simulink model "dl_adaptor"  (R2020b)
settings: Solver=ode45  StartTime=0.0  StopTime=sim_time  RelTol=1e-3  EnableMultiTasking=on
values from neighbouring files (symbols this model uses):
  bw_case = 0    [dl_adaptor_init.m]
  compression_mode = 0    [dl_adaptor_init.m]
  data_bin_pt = 0    [dl_adaptor_init.m]
  data_bit_width = 16    [dl_adaptor_init.m]
  dl_oran_gain_bin_pt = 14    [dl_adaptor_init.m]
  dl_oran_gain_reg = round(dl_oran_gain_reg*2^dl_oran_gain_bin_pt)*2^-dl_oran_gain_bin_pt    [dl_adaptor_init.m]
  eq_gain_bit_width = 9    [dl_adaptor_init.m]
  equalization_bypass = 0    [dl_adaptor_init.m]
  gain_bit_width = 16    [dl_adaptor_init.m]
  IQ_exp_offset = 0    [dl_adaptor_init.m]
  RAT_mode = 0    [dl_adaptor_init.m]
  sys_clk = 491.52e6    (= 491520000)    [dl_adaptor_init.m]
undefined symbols (not defined in the file or in its folder): A, A2, B, D, i, W, X, Z
libraries: xbsIndex_r4 x372
(part 2 of 2)

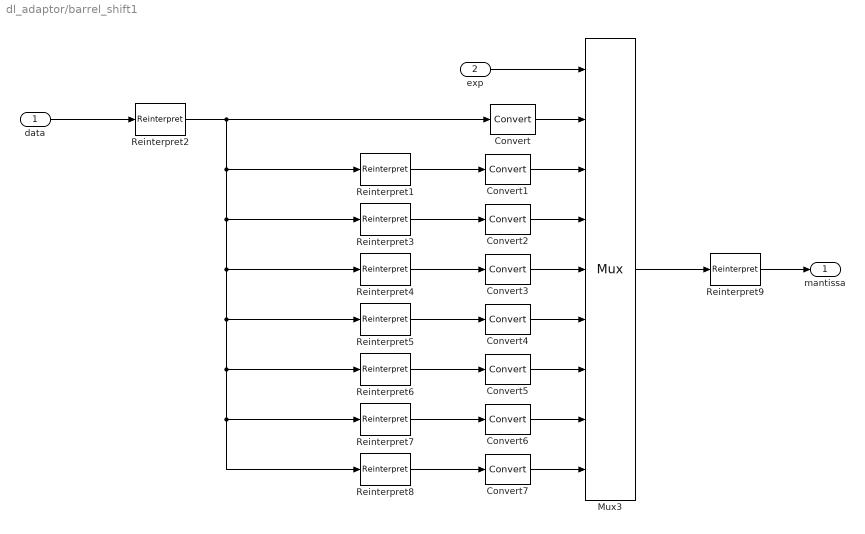
== system dl_adaptor/barrel_shift1 ==
  data : Inport
  exp : Inport  Port=2
  Convert{,1..7} (8 alike) : xbsIndex_r4/Convert  gui_display_data_type=Fixed-point  arith_type="Signed  (2's comp)"  n_bits=data_bit_width  bin_pt=7  float_type=Single  exp_bits=8  fraction_bits=24  quantization=Truncate  overflow=Wrap  en=off  latency=0  pipeline=off  dbl_ovrd=off  block_type=convert
  Mux3 : xbsIndex_r4/Mux  inputs=8  en=off  latency=0  precision=Full  arith_type=Unsigned  n_bits=16  bin_pt=14  quantization=Truncate  overflow=Wrap  dbl_ovrd=off  block_type=mux
  Reinterpret1 : xbsIndex_r4/Reinterpret  force_arith_type=on  arith_type="Signed  (2's comp)"  force_bin_pt=on  bin_pt=6  block_type=reinterpret
  Reinterpret2 : xbsIndex_r4/Reinterpret  force_arith_type=on  arith_type="Signed  (2's comp)"  force_bin_pt=on  bin_pt=7  block_type=reinterpret
  Reinterpret3 : xbsIndex_r4/Reinterpret  force_arith_type=on  arith_type="Signed  (2's comp)"  force_bin_pt=on  bin_pt=5  block_type=reinterpret
  Reinterpret4 : xbsIndex_r4/Reinterpret  force_arith_type=on  arith_type="Signed  (2's comp)"  force_bin_pt=on  bin_pt=4  block_type=reinterpret
  Reinterpret5 : xbsIndex_r4/Reinterpret  force_arith_type=on  arith_type="Signed  (2's comp)"  force_bin_pt=on  bin_pt=3  block_type=reinterpret
  Reinterpret6 : xbsIndex_r4/Reinterpret  force_arith_type=on  arith_type="Signed  (2's comp)"  force_bin_pt=on  bin_pt=2  block_type=reinterpret
  Reinterpret7 : xbsIndex_r4/Reinterpret  force_arith_type=on  arith_type="Signed  (2's comp)"  force_bin_pt=on  bin_pt=1  block_type=reinterpret
  Reinterpret8 : xbsIndex_r4/Reinterpret  force_arith_type=on  arith_type="Signed  (2's comp)"  force_bin_pt=on  bin_pt=0  block_type=reinterpret
  Reinterpret9 : xbsIndex_r4/Reinterpret  force_arith_type=on  arith_type="Signed  (2's comp)"  force_bin_pt=on  bin_pt=0  block_type=reinterpret
  mantissa : Outport  VectorParamsAs1DForOutWhenUnconnected=off
  wires:
  data/1 -> Reinterpret2/1
  Reinterpret1/1 -> Convert1/1
  exp/1 -> Mux3/1
  Mux3/1 -> Reinterpret9/1
  Convert/1 -> Mux3/2
  Convert1/1 -> Mux3/3
  Convert2/1 -> Mux3/4
  Convert3/1 -> Mux3/5
  Convert4/1 -> Mux3/6
  Convert5/1 -> Mux3/7
  Convert6/1 -> Mux3/8
  Reinterpret2/1 -> Convert/1, Reinterpret1/1, Reinterpret3/1, Reinterpret4/1, Reinterpret5/1, Reinterpret6/1, Reinterpret8/1, Reinterpret7/1
  Convert7/1 -> Mux3/9
  Reinterpret3/1 -> Convert2/1
  Reinterpret4/1 -> Convert3/1
  Reinterpret5/1 -> Convert4/1
  Reinterpret6/1 -> Convert5/1
  Reinterpret7/1 -> Convert6/1
  Reinterpret8/1 -> Convert7/1
  Reinterpret9/1 -> mantissa/1

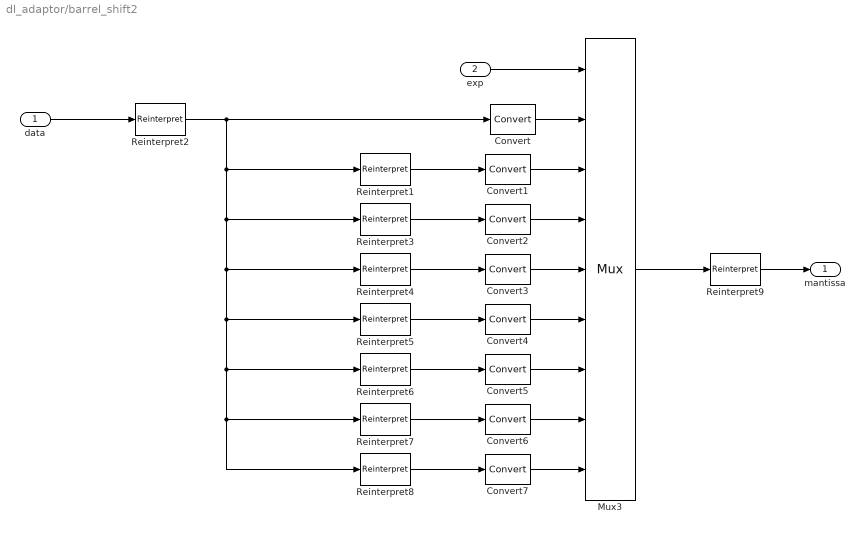
== system dl_adaptor/barrel_shift2 ==
  data : Inport
  exp : Inport  Port=2
  Convert{,1..7} (8 alike) : xbsIndex_r4/Convert  gui_display_data_type=Fixed-point  arith_type="Signed  (2's comp)"  n_bits=data_bit_width  bin_pt=7  float_type=Single  exp_bits=8  fraction_bits=24  quantization=Truncate  overflow=Wrap  en=off  latency=0  pipeline=off  dbl_ovrd=off  block_type=convert
  Mux3 : xbsIndex_r4/Mux  inputs=8  en=off  latency=0  precision=Full  arith_type=Unsigned  n_bits=16  bin_pt=14  quantization=Truncate  overflow=Wrap  dbl_ovrd=off  block_type=mux
  Reinterpret1 : xbsIndex_r4/Reinterpret  force_arith_type=on  arith_type="Signed  (2's comp)"  force_bin_pt=on  bin_pt=6  block_type=reinterpret
  Reinterpret2 : xbsIndex_r4/Reinterpret  force_arith_type=on  arith_type="Signed  (2's comp)"  force_bin_pt=on  bin_pt=7  block_type=reinterpret
  Reinterpret3 : xbsIndex_r4/Reinterpret  force_arith_type=on  arith_type="Signed  (2's comp)"  force_bin_pt=on  bin_pt=5  block_type=reinterpret
  Reinterpret4 : xbsIndex_r4/Reinterpret  force_arith_type=on  arith_type="Signed  (2's comp)"  force_bin_pt=on  bin_pt=4  block_type=reinterpret
  Reinterpret5 : xbsIndex_r4/Reinterpret  force_arith_type=on  arith_type="Signed  (2's comp)"  force_bin_pt=on  bin_pt=3  block_type=reinterpret
  Reinterpret6 : xbsIndex_r4/Reinterpret  force_arith_type=on  arith_type="Signed  (2's comp)"  force_bin_pt=on  bin_pt=2  block_type=reinterpret
  Reinterpret7 : xbsIndex_r4/Reinterpret  force_arith_type=on  arith_type="Signed  (2's comp)"  force_bin_pt=on  bin_pt=1  block_type=reinterpret
  Reinterpret8 : xbsIndex_r4/Reinterpret  force_arith_type=on  arith_type="Signed  (2's comp)"  force_bin_pt=on  bin_pt=0  block_type=reinterpret
  Reinterpret9 : xbsIndex_r4/Reinterpret  force_arith_type=on  arith_type="Signed  (2's comp)"  force_bin_pt=on  bin_pt=0  block_type=reinterpret
  mantissa : Outport  VectorParamsAs1DForOutWhenUnconnected=off
  wires:
  data/1 -> Reinterpret2/1
  Reinterpret1/1 -> Convert1/1
  exp/1 -> Mux3/1
  Mux3/1 -> Reinterpret9/1
  Convert/1 -> Mux3/2
  Convert1/1 -> Mux3/3
  Convert2/1 -> Mux3/4
  Convert3/1 -> Mux3/5
  Convert4/1 -> Mux3/6
  Convert5/1 -> Mux3/7
  Convert6/1 -> Mux3/8
  Reinterpret2/1 -> Convert/1, Reinterpret1/1, Reinterpret3/1, Reinterpret4/1, Reinterpret5/1, Reinterpret6/1, Reinterpret8/1, Reinterpret7/1
  Convert7/1 -> Mux3/9
  Reinterpret3/1 -> Convert2/1
  Reinterpret4/1 -> Convert3/1
  Reinterpret5/1 -> Convert4/1
  Reinterpret6/1 -> Convert5/1
  Reinterpret7/1 -> Convert6/1
  Reinterpret8/1 -> Convert7/1
  Reinterpret9/1 -> mantissa/1

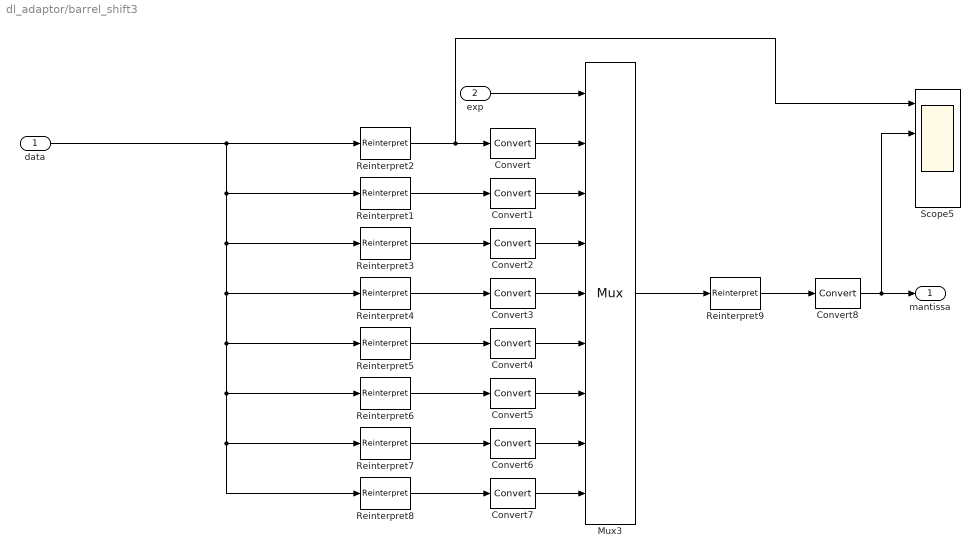
== system dl_adaptor/barrel_shift3 ==
  data : Inport
  exp : Inport  Port=2
  Convert{,1..7} (8 alike) : xbsIndex_r4/Convert  gui_display_data_type=Fixed-point  arith_type=Unsigned  n_bits=gain_bit_width-1  bin_pt=4  float_type=Single  exp_bits=8  fraction_bits=24  quantization=Truncate  overflow=Wrap  en=off  latency=0  pipeline=off  dbl_ovrd=off  block_type=convert
  Convert8 : xbsIndex_r4/Convert  gui_display_data_type=Fixed-point  arith_type="Signed  (2's comp)"  n_bits=gain_bit_width  bin_pt=gain_bin_pt  float_type=Single  exp_bits=8  fraction_bits=24  quantization=Truncate  overflow=Wrap  en=off  latency=0  pipeline=off  dbl_ovrd=off  block_type=convert
  Mux3 : xbsIndex_r4/Mux  inputs=8  en=off  latency=0  precision=Full  arith_type=Unsigned  n_bits=16  bin_pt=14  quantization=Truncate  overflow=Wrap  dbl_ovrd=off  block_type=mux
  Reinterpret1 : xbsIndex_r4/Reinterpret  force_arith_type=on  arith_type=Unsigned  force_bin_pt=on  bin_pt=1  block_type=reinterpret
  Reinterpret2 : xbsIndex_r4/Reinterpret  force_arith_type=on  arith_type=Unsigned  force_bin_pt=on  bin_pt=0  block_type=reinterpret
  Reinterpret3 : xbsIndex_r4/Reinterpret  force_arith_type=on  arith_type=Unsigned  force_bin_pt=on  bin_pt=2  block_type=reinterpret
  Reinterpret4 : xbsIndex_r4/Reinterpret  force_arith_type=on  arith_type=Unsigned  force_bin_pt=on  bin_pt=3  block_type=reinterpret
  Reinterpret5 : xbsIndex_r4/Reinterpret  force_arith_type=on  arith_type=Unsigned  force_bin_pt=on  bin_pt=4  block_type=reinterpret
  Reinterpret6 : xbsIndex_r4/Reinterpret  force_arith_type=on  arith_type=Unsigned  force_bin_pt=on  bin_pt=5  block_type=reinterpret
  Reinterpret7 : xbsIndex_r4/Reinterpret  force_arith_type=on  arith_type=Unsigned  force_bin_pt=on  bin_pt=6  block_type=reinterpret
  Reinterpret8 : xbsIndex_r4/Reinterpret  force_arith_type=on  arith_type=Unsigned  force_bin_pt=on  bin_pt=7  block_type=reinterpret
  Reinterpret9 : xbsIndex_r4/Reinterpret  force_arith_type=on  arith_type=Unsigned  force_bin_pt=on  bin_pt=gain_bit_width-1  block_type=reinterpret
  Scope5 : Scope  NumInputPorts=4
  mantissa : Outport  VectorParamsAs1DForOutWhenUnconnected=off
  wires:
  Reinterpret1/1 -> Convert1/1
  exp/1 -> Mux3/1
  Mux3/1 -> Reinterpret9/1
  Convert/1 -> Mux3/2
  Convert1/1 -> Mux3/3
  Convert2/1 -> Mux3/4
  Convert3/1 -> Mux3/5
  Convert4/1 -> Mux3/6
  Convert5/1 -> Mux3/7
  Convert6/1 -> Mux3/8
  data/1 -> Reinterpret2/1, Reinterpret1/1, Reinterpret3/1, Reinterpret4/1, Reinterpret5/1, Reinterpret6/1, Reinterpret8/1, Reinterpret7/1
  Convert7/1 -> Mux3/9
  Reinterpret3/1 -> Convert2/1
  Reinterpret4/1 -> Convert3/1
  Reinterpret5/1 -> Convert4/1
  Reinterpret6/1 -> Convert5/1
  Reinterpret7/1 -> Convert6/1
  Reinterpret8/1 -> Convert7/1
  Reinterpret9/1 -> Convert8/1
  Reinterpret2/1 -> Scope5/1, Convert/1
  Convert8/1 -> Scope5/2, mantissa/1

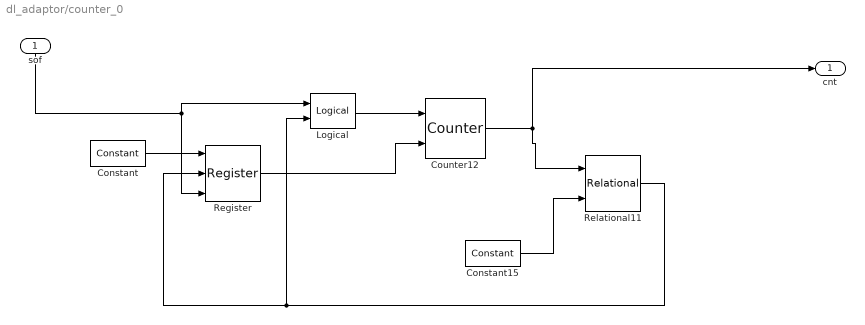
== system dl_adaptor/counter_0 ==
  sof : Inport
  Constant : xbsIndex_r4/Constant  const=1  gui_display_data_type=Boolean  arith_type=Boolean  n_bits=16  bin_pt=14  preci_type=Single  exp_width=8  frac_width=24  explicit_period=off  period=1  equ=P=C  opselect=C  inp2=PCIN>>17  opr=+  inp1=P  carry=CIN  dbl_ovrd=off  block_type=constant
  Constant15 : xbsIndex_r4/Constant  const=2^16-2  gui_display_data_type=Fixed-point  arith_type=Unsigned  n_bits=16  bin_pt=0  preci_type=Single  exp_width=8  frac_width=24  explicit_period=off  period=1  equ=P=C  opselect=C  inp2=PCIN>>17  opr=+  inp1=P  carry=CIN  dbl_ovrd=off  block_type=constant
  Counter12 : xbsIndex_r4/Counter  cnt_type=Free Running  cnt_to=Inf  operation=Up  start_count=0  cnt_by_val=1  arith_type=Unsigned  n_bits=16  bin_pt=0  load_pin=off  rst=on  en=on  explicit_period=on  period=tc  use_behavioral_HDL=off  implementation=Fabric  dbl_ovrd=off  block_type=counter
  Logical : xbsIndex_r4/Logical  logical_function=OR  inputs=2  en=off  latency=0  precision=Full  arith_type=Unsigned  n_bits=16  bin_pt=0  align_bp=on  dbl_ovrd=off  block_type=logical
  Register : xbsIndex_r4/Register  init=0  rst=on  en=on  dbl_ovrd=off  block_type=register
  Relational11 : xbsIndex_r4/Relational  mode=a=b  op_type=Bool  en=off  latency=1  dbl_ovrd=off  block_type=relational
  cnt : Outport  VectorParamsAs1DForOutWhenUnconnected=off
  wires:
  Counter12/1 -> Relational11/1, cnt/1
  Constant15/1 -> Relational11/2
  Register/1 -> Counter12/2
  Constant/1 -> Register/1
  sof/1 -> Logical/1, Register/3
  Logical/1 -> Counter12/1
  Relational11/1 -> Logical/2, Register/2

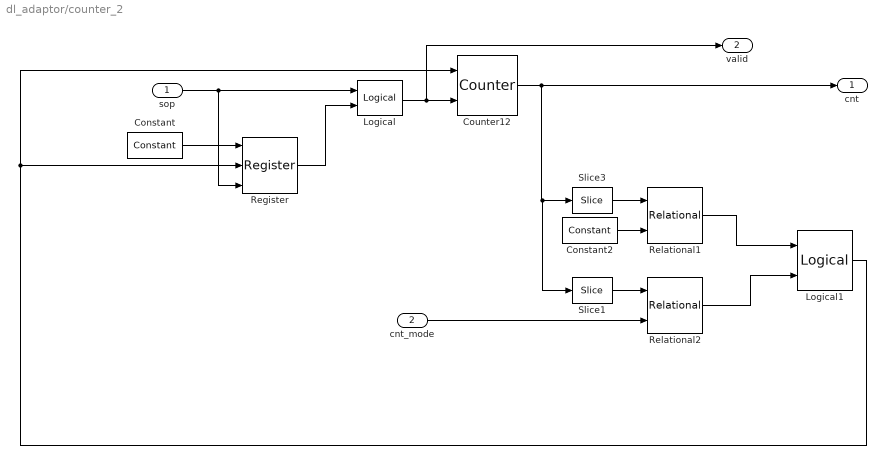
== system dl_adaptor/counter_2 ==
  sop : Inport
  cnt_mode : Inport  Port=2
  Constant : xbsIndex_r4/Constant  const=1  gui_display_data_type=Boolean  arith_type=Boolean  n_bits=16  bin_pt=14  preci_type=Single  exp_width=8  frac_width=24  explicit_period=off  period=1  equ=P=C  opselect=C  inp2=PCIN>>17  opr=+  inp1=P  carry=CIN  dbl_ovrd=off  block_type=constant
  Constant2 : xbsIndex_r4/Constant  const=2^13-2  gui_display_data_type=Fixed-point  arith_type=Unsigned  n_bits=13  bin_pt=0  preci_type=Single  exp_width=8  frac_width=24  explicit_period=off  period=1  equ=P=C  opselect=C  inp2=PCIN>>17  opr=+  inp1=P  carry=CIN  dbl_ovrd=off  block_type=constant
  Counter12 : xbsIndex_r4/Counter  cnt_type=Free Running  cnt_to=Inf  operation=Up  start_count=0  cnt_by_val=1  arith_type=Unsigned  n_bits=15  bin_pt=0  load_pin=off  rst=on  en=on  explicit_period=on  period=tc  use_behavioral_HDL=off  implementation=Fabric  dbl_ovrd=off  block_type=counter
  Logical : xbsIndex_r4/Logical  logical_function=OR  inputs=2  en=off  latency=0  precision=Full  arith_type=Unsigned  n_bits=16  bin_pt=0  align_bp=on  dbl_ovrd=off  block_type=logical
  Logical1 : xbsIndex_r4/Logical  logical_function=AND  inputs=2  en=off  latency=1  precision=Full  arith_type=Unsigned  n_bits=16  bin_pt=0  align_bp=on  dbl_ovrd=off  block_type=logical
  Register : xbsIndex_r4/Register  init=0  rst=on  en=on  dbl_ovrd=off  block_type=register
  Relational1 : xbsIndex_r4/Relational  mode=a=b  op_type=Bool  en=off  latency=0  dbl_ovrd=off  block_type=relational
  Relational2 : xbsIndex_r4/Relational  mode=a=b  op_type=Bool  en=off  latency=0  dbl_ovrd=off  block_type=relational
  Slice1 : xbsIndex_r4/Slice  nbits=2  boolean_output=off  mode=Upper Bit Location + Width  bit1=0  base1=MSB of Input  bit0=0  base0=LSB of Input  dbl_ovrd=off  block_type=slice
  Slice3 : xbsIndex_r4/Slice  nbits=13  boolean_output=off  mode=Lower Bit Location + Width  bit1=0  base1=MSB of Input  bit0=0  base0=LSB of Input  dbl_ovrd=off  block_type=slice
  cnt : Outport  VectorParamsAs1DForOutWhenUnconnected=off
  valid : Outport  Port=2  VectorParamsAs1DForOutWhenUnconnected=off
  wires:
  Slice1/1 -> Relational2/1
  Logical1/1 -> Register/2, Counter12/1
  cnt_mode/1 -> Relational2/2
  Counter12/1 -> Slice1/1, Slice3/1, cnt/1
  Constant2/1 -> Relational1/2
  Register/1 -> Logical/2
  Constant/1 -> Register/1
  Relational2/1 -> Logical1/2
  Slice3/1 -> Relational1/1
  Relational1/1 -> Logical1/1
  sop/1 -> Register/3, Logical/1
  Logical/1 -> valid/1, Counter12/2

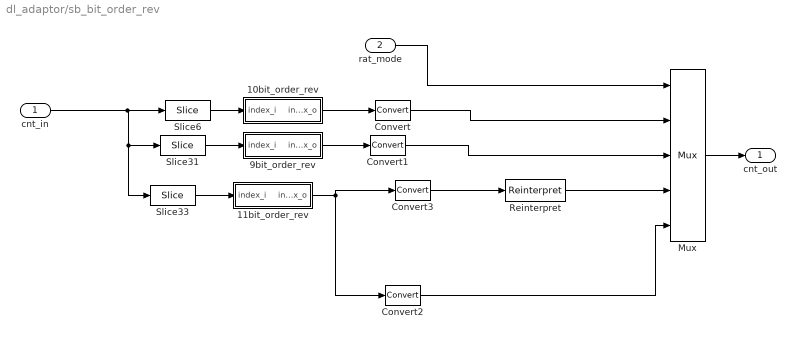
== system dl_adaptor/sb_bit_order_rev ==
  cnt_in : Inport
  rat_mode : Inport  Port=2
  10bit_order_rev : Subsystem
  11bit_order_rev : Subsystem
  9bit_order_rev : Subsystem
  Convert : xbsIndex_r4/Convert  gui_display_data_type=Fixed-point  arith_type=Unsigned  n_bits=12  bin_pt=0  float_type=Single  exp_bits=8  fraction_bits=24  quantization=Truncate  overflow=Wrap  en=off  latency=0  pipeline=off  dbl_ovrd=off  block_type=convert
  Convert1 : xbsIndex_r4/Convert  gui_display_data_type=Fixed-point  arith_type=Unsigned  n_bits=12  bin_pt=0  float_type=Single  exp_bits=8  fraction_bits=24  quantization=Truncate  overflow=Wrap  en=off  latency=0  pipeline=off  dbl_ovrd=off  block_type=convert
  Convert2 : xbsIndex_r4/Convert  gui_display_data_type=Fixed-point  arith_type=Unsigned  n_bits=12  bin_pt=0  float_type=Single  exp_bits=8  fraction_bits=24  quantization=Truncate  overflow=Wrap  en=off  latency=0  pipeline=off  dbl_ovrd=off  block_type=convert
  Convert3 : xbsIndex_r4/Convert  gui_display_data_type=Fixed-point  arith_type=Unsigned  n_bits=12  bin_pt=1  float_type=Single  exp_bits=8  fraction_bits=24  quantization=Truncate  overflow=Wrap  en=off  latency=0  pipeline=off  dbl_ovrd=off  block_type=convert
  Mux : xbsIndex_r4/Mux  inputs=4  en=off  latency=0  precision=Full  arith_type=Unsigned  n_bits=16  bin_pt=14  quantization=Truncate  overflow=Wrap  dbl_ovrd=off  block_type=mux
  Reinterpret : xbsIndex_r4/Reinterpret  force_arith_type=on  arith_type=Unsigned  force_bin_pt=on  bin_pt=0  block_type=reinterpret
  Slice31 : xbsIndex_r4/Slice  nbits=9  boolean_output=off  mode=Upper Bit Location + Width  bit1=-2  base1=MSB of Input  bit0=0  base0=LSB of Input  dbl_ovrd=off  block_type=slice
  Slice33 : xbsIndex_r4/Slice  nbits=11  boolean_output=off  mode=Upper Bit Location + Width  bit1=0  base1=MSB of Input  bit0=0  base0=LSB of Input  dbl_ovrd=off  block_type=slice
  Slice6 : xbsIndex_r4/Slice  nbits=10  boolean_output=off  mode=Upper Bit Location + Width  bit1=-1  base1=MSB of Input  bit0=0  base0=LSB of Input  dbl_ovrd=off  block_type=slice
  cnt_out : Outport  VectorParamsAs1DForOutWhenUnconnected=off
  wires:
  10bit_order_rev/1(index_o) -> Convert/1
  Slice33/1 -> 11bit_order_rev/1(index_i)
  Slice6/1 -> 10bit_order_rev/1(index_i)
  Slice31/1 -> 9bit_order_rev/1(index_i)
  cnt_in/1 -> Slice6/1, Slice33/1, Slice31/1
  11bit_order_rev/1(index_o) -> Convert3/1, Convert2/1
  9bit_order_rev/1(index_o) -> Convert1/1
  rat_mode/1 -> Mux/1
  Convert/1 -> Mux/2
  Convert1/1 -> Mux/3
  Mux/1 -> cnt_out/1
  Convert2/1 -> Mux/5
  Convert3/1 -> Reinterpret/1
  Reinterpret/1 -> Mux/4

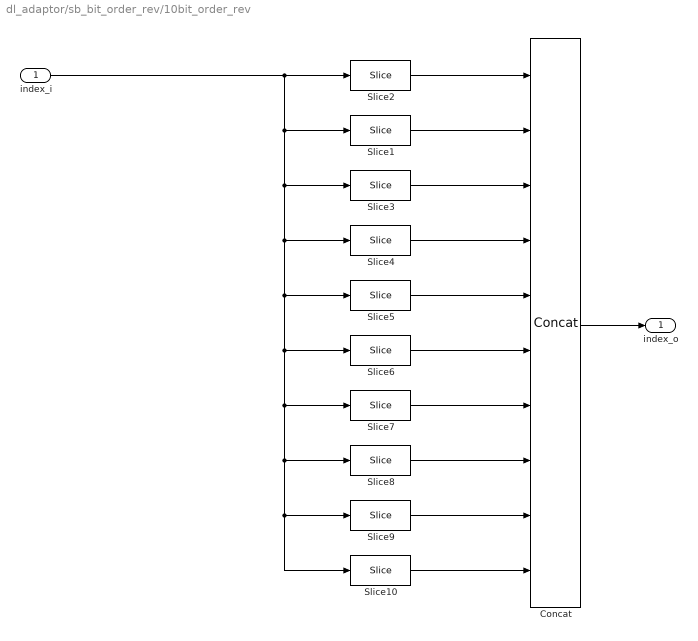
== system dl_adaptor/sb_bit_order_rev/10bit_order_rev ==
  index_i : Inport
  Concat : xbsIndex_r4/Concat  num_inputs=10  dbl_ovrd=off  block_type=concat
  Slice1 : xbsIndex_r4/Slice  nbits=1  boolean_output=off  mode=Lower Bit Location + Width  bit1=0  base1=MSB of Input  bit0=1  base0=LSB of Input  dbl_ovrd=off  block_type=slice
  Slice10 : xbsIndex_r4/Slice  nbits=1  boolean_output=off  mode=Lower Bit Location + Width  bit1=0  base1=MSB of Input  bit0=9  base0=LSB of Input  dbl_ovrd=off  block_type=slice
  Slice2 : xbsIndex_r4/Slice  nbits=1  boolean_output=off  mode=Lower Bit Location + Width  bit1=0  base1=MSB of Input  bit0=0  base0=LSB of Input  dbl_ovrd=off  block_type=slice
  Slice3 : xbsIndex_r4/Slice  nbits=1  boolean_output=off  mode=Lower Bit Location + Width  bit1=0  base1=MSB of Input  bit0=2  base0=LSB of Input  dbl_ovrd=off  block_type=slice
  Slice4 : xbsIndex_r4/Slice  nbits=1  boolean_output=off  mode=Lower Bit Location + Width  bit1=0  base1=MSB of Input  bit0=3  base0=LSB of Input  dbl_ovrd=off  block_type=slice
  Slice5 : xbsIndex_r4/Slice  nbits=1  boolean_output=off  mode=Lower Bit Location + Width  bit1=0  base1=MSB of Input  bit0=4  base0=LSB of Input  dbl_ovrd=off  block_type=slice
  Slice6 : xbsIndex_r4/Slice  nbits=1  boolean_output=off  mode=Lower Bit Location + Width  bit1=0  base1=MSB of Input  bit0=5  base0=LSB of Input  dbl_ovrd=off  block_type=slice
  Slice7 : xbsIndex_r4/Slice  nbits=1  boolean_output=off  mode=Lower Bit Location + Width  bit1=0  base1=MSB of Input  bit0=6  base0=LSB of Input  dbl_ovrd=off  block_type=slice
  Slice8 : xbsIndex_r4/Slice  nbits=1  boolean_output=off  mode=Lower Bit Location + Width  bit1=0  base1=MSB of Input  bit0=7  base0=LSB of Input  dbl_ovrd=off  block_type=slice
  Slice9 : xbsIndex_r4/Slice  nbits=1  boolean_output=off  mode=Lower Bit Location + Width  bit1=0  base1=MSB of Input  bit0=8  base0=LSB of Input  dbl_ovrd=off  block_type=slice
  index_o : Outport  VectorParamsAs1DForOutWhenUnconnected=off
  wires:
  index_i/1 -> Slice1/1, Slice3/1, Slice4/1, Slice5/1, Slice6/1, Slice7/1, Slice8/1, Slice9/1, Slice10/1, Slice2/1
  Slice2/1 -> Concat/1
  Concat/1 -> index_o/1
  Slice1/1 -> Concat/2
  Slice10/1 -> Concat/10
  Slice7/1 -> Concat/7
  Slice3/1 -> Concat/3
  Slice8/1 -> Concat/8
  Slice9/1 -> Concat/9
  Slice6/1 -> Concat/6
  Slice5/1 -> Concat/5
  Slice4/1 -> Concat/4

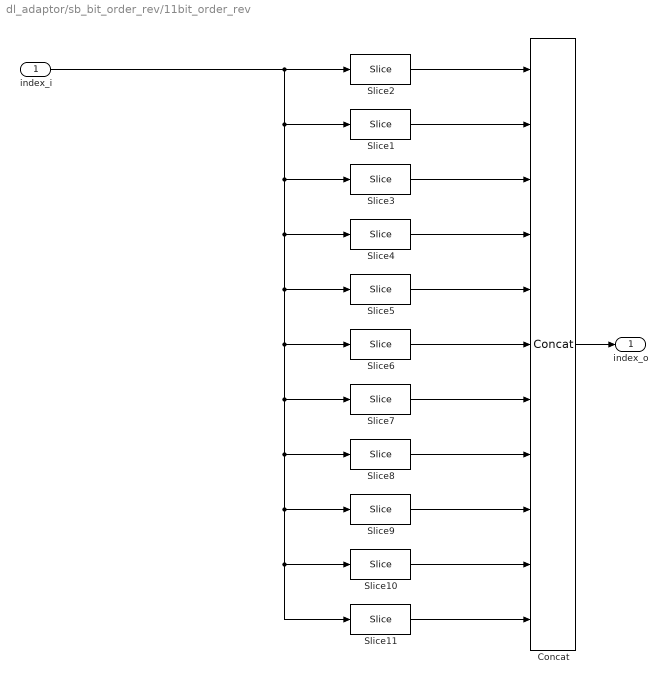
== system dl_adaptor/sb_bit_order_rev/11bit_order_rev ==
  index_i : Inport
  Concat : xbsIndex_r4/Concat  num_inputs=11  dbl_ovrd=off  block_type=concat
  Slice1 : xbsIndex_r4/Slice  nbits=1  boolean_output=off  mode=Lower Bit Location + Width  bit1=0  base1=MSB of Input  bit0=1  base0=LSB of Input  dbl_ovrd=off  block_type=slice
  Slice10 : xbsIndex_r4/Slice  nbits=1  boolean_output=off  mode=Lower Bit Location + Width  bit1=0  base1=MSB of Input  bit0=9  base0=LSB of Input  dbl_ovrd=off  block_type=slice
  Slice11 : xbsIndex_r4/Slice  nbits=1  boolean_output=off  mode=Lower Bit Location + Width  bit1=0  base1=MSB of Input  bit0=10  base0=LSB of Input  dbl_ovrd=off  block_type=slice
  Slice2 : xbsIndex_r4/Slice  nbits=1  boolean_output=off  mode=Lower Bit Location + Width  bit1=0  base1=MSB of Input  bit0=0  base0=LSB of Input  dbl_ovrd=off  block_type=slice
  Slice3 : xbsIndex_r4/Slice  nbits=1  boolean_output=off  mode=Lower Bit Location + Width  bit1=0  base1=MSB of Input  bit0=2  base0=LSB of Input  dbl_ovrd=off  block_type=slice
  Slice4 : xbsIndex_r4/Slice  nbits=1  boolean_output=off  mode=Lower Bit Location + Width  bit1=0  base1=MSB of Input  bit0=3  base0=LSB of Input  dbl_ovrd=off  block_type=slice
  Slice5 : xbsIndex_r4/Slice  nbits=1  boolean_output=off  mode=Lower Bit Location + Width  bit1=0  base1=MSB of Input  bit0=4  base0=LSB of Input  dbl_ovrd=off  block_type=slice
  Slice6 : xbsIndex_r4/Slice  nbits=1  boolean_output=off  mode=Lower Bit Location + Width  bit1=0  base1=MSB of Input  bit0=5  base0=LSB of Input  dbl_ovrd=off  block_type=slice
  Slice7 : xbsIndex_r4/Slice  nbits=1  boolean_output=off  mode=Lower Bit Location + Width  bit1=0  base1=MSB of Input  bit0=6  base0=LSB of Input  dbl_ovrd=off  block_type=slice
  Slice8 : xbsIndex_r4/Slice  nbits=1  boolean_output=off  mode=Lower Bit Location + Width  bit1=0  base1=MSB of Input  bit0=7  base0=LSB of Input  dbl_ovrd=off  block_type=slice
  Slice9 : xbsIndex_r4/Slice  nbits=1  boolean_output=off  mode=Lower Bit Location + Width  bit1=0  base1=MSB of Input  bit0=8  base0=LSB of Input  dbl_ovrd=off  block_type=slice
  index_o : Outport  VectorParamsAs1DForOutWhenUnconnected=off
  wires:
  index_i/1 -> Slice1/1, Slice3/1, Slice4/1, Slice5/1, Slice6/1, Slice7/1, Slice8/1, Slice11/1, Slice10/1, Slice9/1, Slice2/1
  Slice2/1 -> Concat/1
  Concat/1 -> index_o/1
  Slice1/1 -> Concat/2
  Slice7/1 -> Concat/7
  Slice3/1 -> Concat/3
  Slice8/1 -> Concat/8
  Slice9/1 -> Concat/9
  Slice6/1 -> Concat/6
  Slice5/1 -> Concat/5
  Slice4/1 -> Concat/4
  Slice10/1 -> Concat/10
  Slice11/1 -> Concat/11

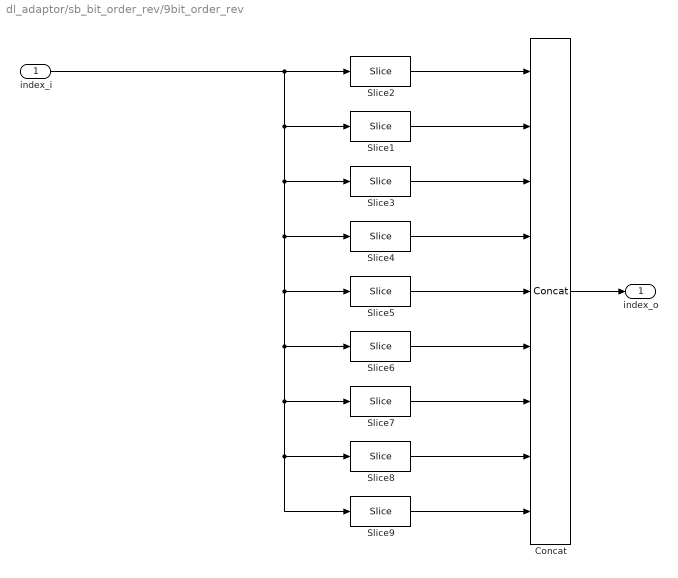
== system dl_adaptor/sb_bit_order_rev/9bit_order_rev ==
  index_i : Inport
  Concat : xbsIndex_r4/Concat  num_inputs=9  dbl_ovrd=off  block_type=concat
  Slice1 : xbsIndex_r4/Slice  nbits=1  boolean_output=off  mode=Lower Bit Location + Width  bit1=0  base1=MSB of Input  bit0=1  base0=LSB of Input  dbl_ovrd=off  block_type=slice
  Slice2 : xbsIndex_r4/Slice  nbits=1  boolean_output=off  mode=Lower Bit Location + Width  bit1=0  base1=MSB of Input  bit0=0  base0=LSB of Input  dbl_ovrd=off  block_type=slice
  Slice3 : xbsIndex_r4/Slice  nbits=1  boolean_output=off  mode=Lower Bit Location + Width  bit1=0  base1=MSB of Input  bit0=2  base0=LSB of Input  dbl_ovrd=off  block_type=slice
  Slice4 : xbsIndex_r4/Slice  nbits=1  boolean_output=off  mode=Lower Bit Location + Width  bit1=0  base1=MSB of Input  bit0=3  base0=LSB of Input  dbl_ovrd=off  block_type=slice
  Slice5 : xbsIndex_r4/Slice  nbits=1  boolean_output=off  mode=Lower Bit Location + Width  bit1=0  base1=MSB of Input  bit0=4  base0=LSB of Input  dbl_ovrd=off  block_type=slice
  Slice6 : xbsIndex_r4/Slice  nbits=1  boolean_output=off  mode=Lower Bit Location + Width  bit1=0  base1=MSB of Input  bit0=5  base0=LSB of Input  dbl_ovrd=off  block_type=slice
  Slice7 : xbsIndex_r4/Slice  nbits=1  boolean_output=off  mode=Lower Bit Location + Width  bit1=0  base1=MSB of Input  bit0=6  base0=LSB of Input  dbl_ovrd=off  block_type=slice
  Slice8 : xbsIndex_r4/Slice  nbits=1  boolean_output=off  mode=Lower Bit Location + Width  bit1=0  base1=MSB of Input  bit0=7  base0=LSB of Input  dbl_ovrd=off  block_type=slice
  Slice9 : xbsIndex_r4/Slice  nbits=1  boolean_output=off  mode=Lower Bit Location + Width  bit1=0  base1=MSB of Input  bit0=8  base0=LSB of Input  dbl_ovrd=off  block_type=slice
  index_o : Outport  VectorParamsAs1DForOutWhenUnconnected=off
  wires:
  index_i/1 -> Slice1/1, Slice3/1, Slice4/1, Slice5/1, Slice6/1, Slice7/1, Slice8/1, Slice9/1, Slice2/1
  Slice2/1 -> Concat/1
  Concat/1 -> index_o/1
  Slice1/1 -> Concat/2
  Slice7/1 -> Concat/7
  Slice3/1 -> Concat/3
  Slice8/1 -> Concat/8
  Slice9/1 -> Concat/9
  Slice6/1 -> Concat/6
  Slice5/1 -> Concat/5
  Slice4/1 -> Concat/4
